simulink model "w1p3"  (R2020b)
settings: Solver=VariableStepAuto  StartTime=0.0  StopTime=10.0  RelTol=1e-3
settings Model: Creator=WELCOME  LastModifiedBy=WELCOME

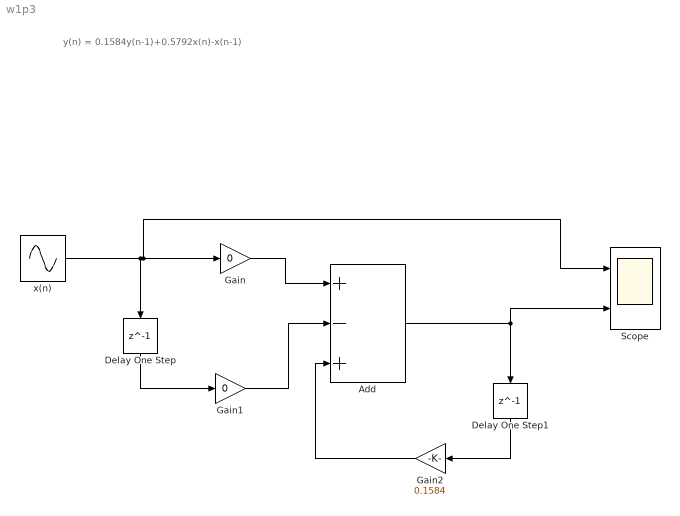
== system w1p3 ==
  note: y(n) = 0.1584y(n-1)+0.5792x(n)-x(n-1)
  Add : Sum  Inputs=+-+
  Delay One Step : Delay  DelayLength=1
  Delay One Step1 : Delay  DelayLength=1
  Gain : Gain  Gain=0
  Gain1 : Gain  Gain=0
  Gain2 : Gain  Gain=0.1584
  Scope : Scope  NumInputPorts=2
  x(n) : Sin  Frequency=200  SampleTime=1/5000
  wires:
  Gain/1 -> Add/1
  Gain1/1 -> Add/2
  Delay One Step/1 -> Gain1/1
  Gain2/1 -> Add/3
  Delay One Step1/1 -> Gain2/1
  Add/1 -> Delay One Step1/1, Scope/2
  x(n)/1 -> Scope/1, Gain/1, Delay One Step/1
